simulink model "FF_simulink"  (R2018b)
settings: Solver=VariableStepAuto  StartTime=0.0  StopTime=50  RelTol=1e-3
values from neighbouring files (symbols this model uses):
  alpha = [-10 -9.5 -9 -8.5 -8 -7.5 -7 -6.5 -6 -5.5 -5 -4.5 ... (132 elements, 132x1)]    [Coeficientes.mat]
  CL = [-1.072056 -1.06528 -1.047066 -1.026643 -1.009407 -0.9886886 -0.9605278 -0.9330248 -0.9046997 -0.8327878 -0.7485972 -0.6673373 ... (132 elements, 132x1)]    [Coeficientes.mat]
  Cm = [-0.059 -0.054 -0.065 -0.067 -0.062]    [Coeficientes.mat]
  g = 9.8    [Coeficientes.mat]
  Iyy = 0.0191    [Coeficientes.mat]
  m = 0.8    [Coeficientes.mat]
  V = 15    [Coeficientes.mat]
settings Model: Creator=ferra  LastModifiedBy=ferra

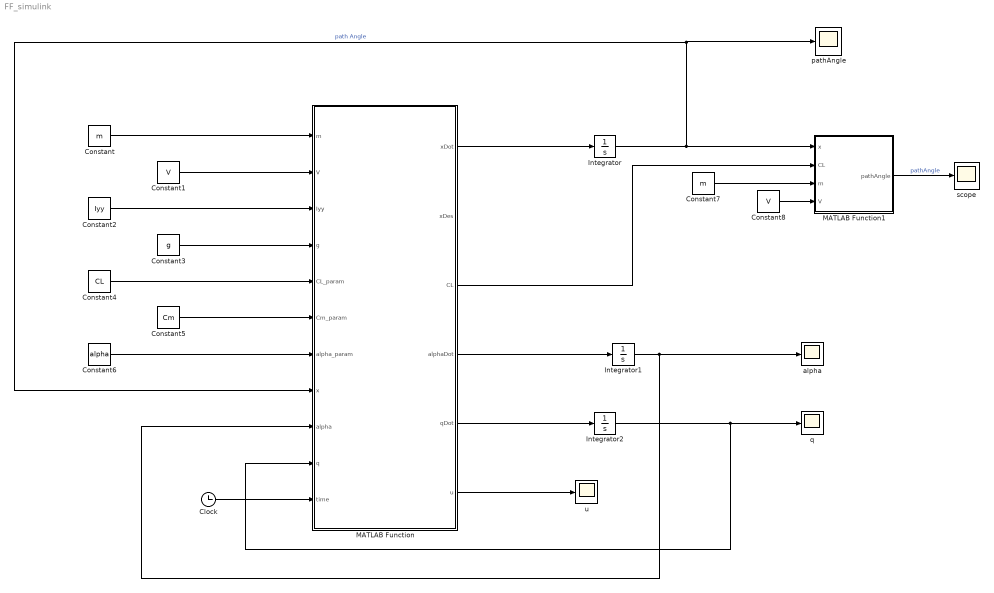
== system FF_simulink ==
  Clock : Clock
  Constant : Constant  Value=m
  Constant1 : Constant  Value=V
  Constant2 : Constant  Value=Iyy
  Constant3 : Constant  Value=g
  Constant4 : Constant  Value=CL
  Constant5 : Constant  Value=Cm
  Constant6 : Constant  Value=alpha
  Constant7 : Constant  Value=m
  Constant8 : Constant  Value=V
  Integrator : Integrator
  Integrator1 : Integrator
  Integrator2 : Integrator
  MATLAB Function : MATLAB Function  TreatAsAtomicUnit=on
  MATLAB Function1 : MATLAB Function  TreatAsAtomicUnit=on
  alpha : Scope
  pathAngle : Scope
  q : Scope
  "scope " : Scope
  u : Scope
  wires:
  Constant/1 -> MATLAB Function/1(m)
  Constant1/1 -> MATLAB Function/2(V)
  Constant2/1 -> MATLAB Function/3(Iyy)
  Constant3/1 -> MATLAB Function/4(g)
  Constant4/1 -> MATLAB Function/5(CL_param)
  Constant5/1 -> MATLAB Function/6(Cm_param)
  MATLAB Function/1(xDot) -> Integrator/1
  MATLAB Function/4(alphaDot) -> Integrator1/1
  MATLAB Function/5(qDot) -> Integrator2/1
  Integrator/1 -> MATLAB Function1/1(x), pathAngle/1, MATLAB Function/8(x)  "path Angle"
  Integrator1/1 -> alpha/1, MATLAB Function/9(alpha)
  Integrator2/1 -> q/1, MATLAB Function/10(q)
  Constant6/1 -> MATLAB Function/7(alpha_param)
  MATLAB Function/6(u) -> u/1
  Constant7/1 -> MATLAB Function1/3(m)
  Constant8/1 -> MATLAB Function1/4(V)
  MATLAB Function/3(CL) -> MATLAB Function1/2(CL)
  MATLAB Function1/1(pathAngle) -> "scope "/1  "pathAngle"
  Clock/1 -> MATLAB Function/11(time)

== matlab function FF_simulink/MATLAB Function1 ==
  data: x input; pathAngle output; CL input; m input; V input
function pathAngle = fromXtoPathAngle(x,CL,m,V)


pathAngle = CL * x/(m*V);
end

== matlab function FF_simulink/MATLAB Function ==
  data: m input; xDot output; xDes output; CL output; V input; Iyy input; g input; CL_param input; Cm_param input; alpha_param input; alphaDot output; qDot output; x input; alpha input; q input; u output; time input
function [xDot,xDes,CL,alphaDot,qDot,u ] = fcn(m,V,Iyy,g,CL_param,Cm_param,...
                                    alpha_param,x,alpha,q,time)
Cm = mean(Cm_param);

k1 = 2;
k2 = 2;

if(alpha>71)
    alpha = 71;
elseif(alpha<-10)
    alpha = -10;
end



alphaRound = round(alpha*2)/2;

seqIndex = 1:1:length(alpha_param);
index = round(interp1(alpha_param,seqIndex,alphaRound));
CL = CL_param(index);

f = (-g/V) * cos((CL*x)/(m*V));
f1 = (g/V) * cos((CL*x)/(m*V)) - (CL*alpha)/(m*V);
f2 = 0;
g2 = Cm/Iyy;



df_dx =( (g*CL)/(m*V^2) ) * sin((CL*x)/(m*V));
df1_dx = ((-g*CL)/(m*V^2) ) *sin((CL*x)/(m*V));
df_ddx = ((g*CL^2)/(m*V^3)) * cos((CL * x)/(m*V));

%Definition of the xDes
amp = 3;
freq = 2*pi/10;
xDes = amp * sin(freq*time);

xDes = 3;

e = x-xDes;
xDesDot = amp *cos(freq*time);
xDesDot = 0;
alphaDes = -f - k1*e + xDesDot; %Virtual : stabilaize the dynamics of x 
alphaDesDot = (-df_dx -k1)*(f+alpha);


e1 = alpha - alphaDes;
qDes = -f1 -x+xDes - k1*e1 + alphaDesDot; %Virtual: stabilize the dynamics of alpha

e2 = q - qDes;

e1Dot = -e - k1*e1 +e2;





d_alphaDesDot_dx = -df_ddx *f - (df_dx)^2 -df_ddx * alpha - k1*df_dx;
par_qDes_x = -df1_dx - 1 + d_alphaDesDot_dx;
par_qDes_e1 = -k1;
qDesDot = par_qDes_x * (f+alpha) + par_qDes_e1 * (e1Dot);
u = (-f2 + qDesDot - e1 - k2*e2)/(g2);

xDot = f + alpha;
alphaDot = f1 + q;
qDot = f2 + g2 *u;
end
